simulink model "replay_example"  (R2024a)
settings: Solver=FixedStepAuto  StartTime=0.0  StopTime=10.0  FixedStep=0.001  RelTol=1e-3
libraries: simulink x1
settings Model: Creator=autod  LastModifiedBy=autod
settings DebuggingCC: UnderspecifiedInitializationDetection=Classic  FrameProcessingCompatibilityMsg=none

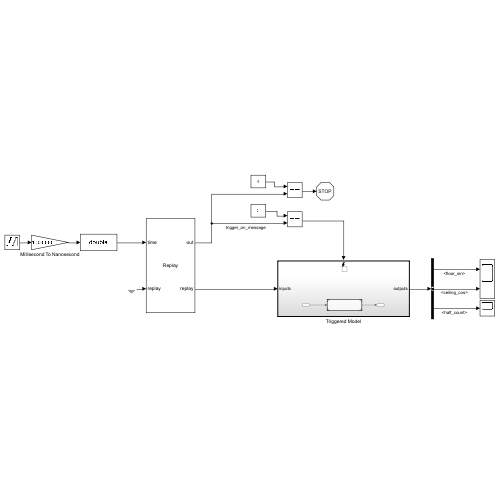
[thumbnail: Simulink's stored preview of the top-level diagram]
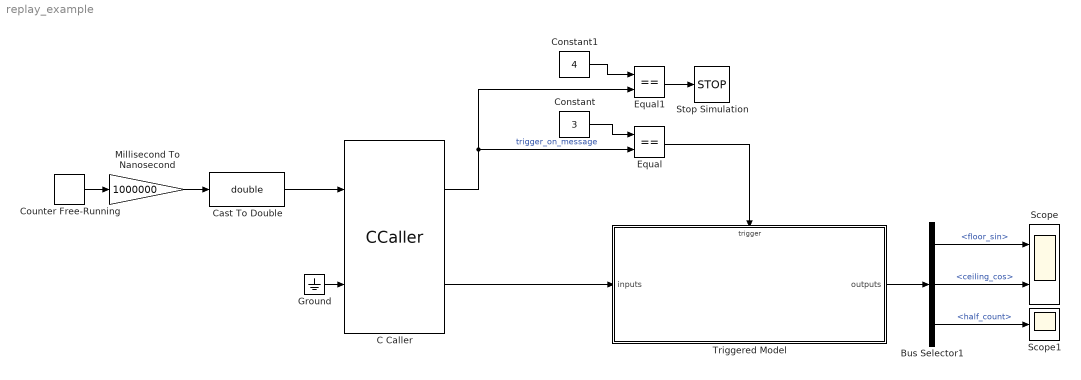
== system replay_example ==
  Bus Selector1 : BusSelector  OutputSignals=floor_sin,ceiling_cos,half_count
  C Caller : CCaller  FunctionName=Replay  PortSpecificationStruct="%)30     .    B 4   8    (     @         %    \"     ,    !     0         %  0 \"0    $    _    07)G3F%M90  4&]R=$YA;64 4V-O<&4     26YD97@     5'EP90      4VEZ90      27-';&]B86P   X    P    !@    @    $          4    (     0    ,    !         !   P!O=70 #@   #     &    \"     0         !0    @    !     P    $         $  # &]U=  .    .     8    (    !          %    \"     $    &     0         0    !@   $]U='!U=   #@   #@    &    \"     8         !0    @    !     0    $         \"0    @               X    X    !@    @    $          4    (     0    <    !         !     '    8F]O;&5A;@ .    ,     8    (    !          %    \"     $    !     0         0  $ ,0    X    P    !@    @    ) @        4    (     0    $    !          (  0      #@   #     &    \"     0         !0    @    !    !     $         $  $ '1I;64.    ,     8    (    !          %    \"     $    $     0         0  0 =&EM90X    X    !@    @    $          4    (     0    4    !         !     %    26YP=70    .    .     8    (    !@         %    \"     $    !     0         )    \"               #@   #@    &    \"     0         !0    @    !    !@    $         $     8   !D;W5B;&4   X    P    !@    @    $          4    (     0    $    !         !   0 Q    #@   #     &    \"     D\"        !0    @    !     0    $          @ !       .    .     8    (    !          %    \"     $    &     0         0    !@   ')E<&QA>0  #@   #@    &    \"     0         !0    @    !    !@    $         $     8   !R97!L87D   X   !     !@    @    $          4    (     0    L    !         !     +    26YP=71/=71P=70       X    X    !@    @    &          4    (     0    $    !          D    (            \\#\\.    4     8    (    !          %    \"     $    ;     0         0    &P   $)U<SH@0G5S7TES;VQA=&5D0V]N=')O;'-)3P      #@   #     &    \"     0         !0    @    !     @    $         $  \" \"TQ   .    ,     8    (    \"0(        %    \"     $    !     0         \"  $"
  Cast To Double : DataTypeConversion  OutDataTypeStr=double  SaturateOnIntegerOverflow=off  RndMeth=Floor
  Constant : Constant  Value=3  OutDataTypeStr=Inherit: Inherit via back propagation
  Constant1 : Constant  Value=4  OutDataTypeStr=Inherit: Inherit via back propagation
  Counter Free-Running : simulink/Sources/Counter Free-Running  NumBits=64  tsamp=-1
  Equal : RelationalOperator  Operator===  OutDataTypeStr=boolean  RndMeth=Simplest  InputSameDT=off
  Equal1 : RelationalOperator  Operator===  OutDataTypeStr=boolean  RndMeth=Simplest  InputSameDT=off
  Ground : Ground
  Millisecond To Nanosecond : Gain  Gain=1000000  OutDataTypeStr=uint64
  Scope : Scope  NumInputPorts=2
  Scope1 : Scope
  Stop Simulation : Stop
  Triggered Model : Subsystem  TreatAsAtomicUnit=on
  wires:
  C Caller/2 -> Triggered Model/1(inputs)
  Millisecond To Nanosecond/1 -> Cast To Double/1
  Ground/1 -> C Caller/2
  Counter Free-Running/1 -> Millisecond To Nanosecond/1
  Constant/1 -> Equal/1
  Equal/1 -> Triggered Model/Trigger
  Equal1/1 -> Stop Simulation/1
  Constant1/1 -> Equal1/1
  C Caller/1 -> Equal/2, Equal1/2  "trigger_on_message"
  Triggered Model/1(outputs) -> Bus Selector1/1
  Bus Selector1/1 -> Scope/1  "<floor_sin>"
  Cast To Double/1 -> C Caller/1
  Bus Selector1/2 -> Scope/2  "<ceiling_cos>"
  Bus Selector1/3 -> Scope1/1  "<half_count>"

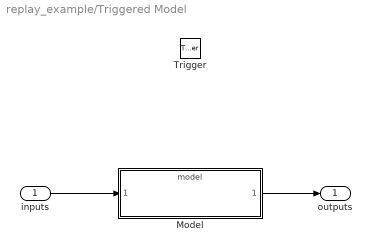
== system replay_example/Triggered Model ==
  inputs : Inport
  Trigger : TriggerPort  VariantControl=(inherit)
  Model : ModelReference  ModelNameDialog=model.slx  SimulationMode=Normal  ModelReferenceVersion=4.59
  outputs : Outport
  wires:
  inputs/1 -> Model/1
  Model/1 -> outputs/1
